simulink model "Mostar_AVR"  (Simulink 10.1)
settings: Solver=VariableStepAuto  StartTime=0  StopTime=6  FixedStep=0.01  RelTol=0.001  EnableMultiTasking=on
libraries: fmu_me_lib x1
settings Model: Creator=Tin Rabuzin  LastModifiedBy=podlam
settings DataIOCC: LimitDataPoints=on  OutputSaveName=simout  OutputOption=SpecifiedOutputTimes  OutputTimes=[0:0.005:6]
settings OptimizationCC: ExpressionDepthLimit=2147483647
settings DebuggingCC: SolverPrmCheckMsg=warning  StateNameClashWarn=warning
settings GRTTargetCC: CombineOutputUpdateFcns=on  GRTInterface=off

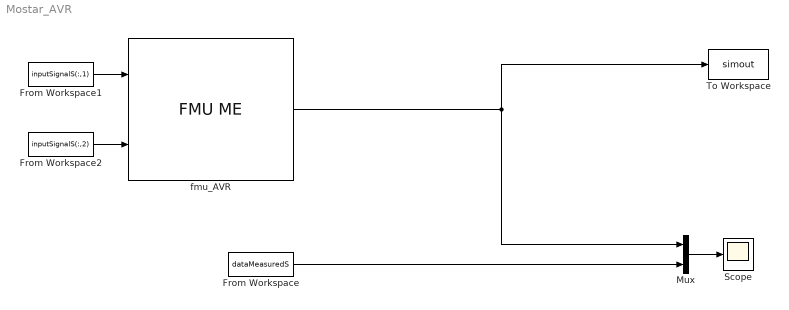
== system Mostar_AVR ==
  From Workspace1 : FromWorkspace  VariableName=inputSignalS(:,1)
  From Workspace2 : FromWorkspace  VariableName=inputSignalS(:,2)
  From Workspace : FromWorkspace  VariableName=dataMeasuredS
  Mux : Mux  Inputs=2
  Scope : Scope
  To Workspace : ToWorkspace  VariableName=simout  SaveFormat=Structure With Time  SampleTime=-1
  fmu_AVR : fmu_me_lib/FMU ME  Description=Simulates an FMU for Model Exchange 1.0 or Model Exchange 2.0.  dummy=0
  wires:
  From Workspace/1 -> Mux/2
  Mux/1 -> Scope/1
  fmu_AVR/1 -> To Workspace/1, Mux/1
  From Workspace1/1 -> fmu_AVR/1
  From Workspace2/1 -> fmu_AVR/2
